simulink subsystem "V2ISimulator"  (R2024a)
settings: Solver=VariableStepAuto  StartTime=0.0  StopTime=10.0  RelTol=1e-3
undefined symbols (not defined in the file or in its folder): SF_std, Ts
settings Model: Creator=The MathWorks, Inc.  LastModifiedBy=L03509110
settings SolverCC: MaxZcPerStep=1
settings DebuggingCC: SubsystemReferenceDiagnosticForUnitTest=warning
settings ModelReferenceCC: EnableRefExpFcnMdlSchedulingChecks=on
settings RTWCC: GPUComputeCapability=3.5  DLArmComputeVersion=19.05

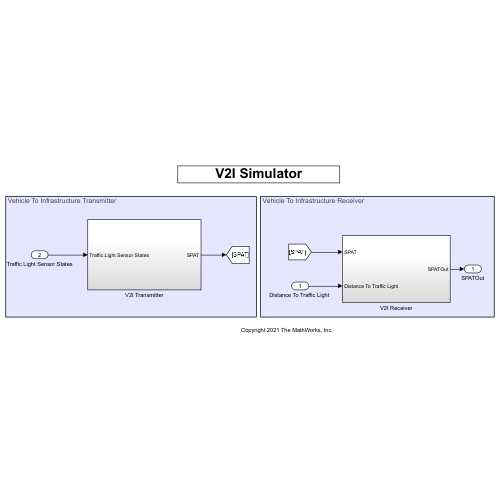
[thumbnail: Simulink's stored preview of the top-level diagram]
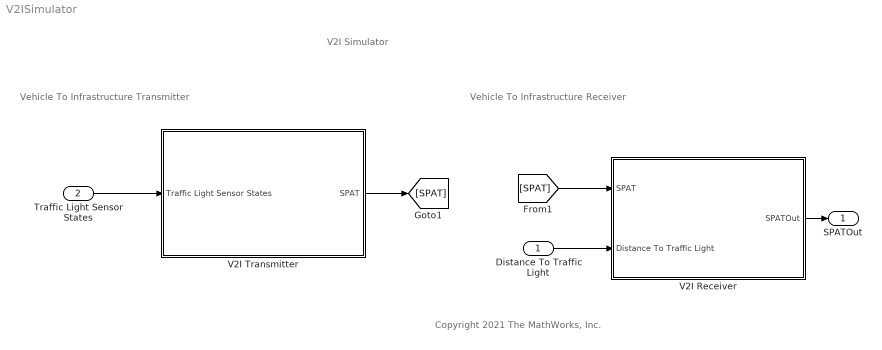
== system V2ISimulator ==
  note: V2I Simulator
  note: Vehicle To Infrastructure Transmitter
  note: Vehicle To Infrastructure Receiver
  note: Copyright 2021 The MathWorks, Inc.
  "Distance To Traffic Light " : Inport
  Traffic Light Sensor States : Inport  Port=2
  V2I Receiver : Subsystem
  V2I Transmitter : Subsystem
  SPATOut : Outport
  wires:
  Traffic Light Sensor States/1 -> V2I Transmitter/1(Traffic Light Sensor States)
  V2I Transmitter/1(SPAT) -> [SPAT]
  V2I Receiver/1(SPATOut) -> SPATOut/1
  "Distance To Traffic Light "/1 -> V2I Receiver/2("Distance To Traffic Light ")
  [SPAT] -> V2I Receiver/1(SPAT)

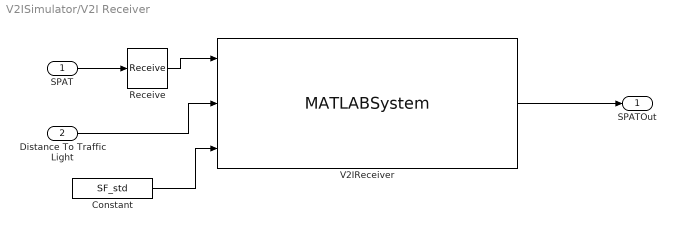
== system V2ISimulator/V2I Receiver ==
  SPAT : Inport  OutDataTypeStr=Bus: BusSPAT  BusOutputAsStruct=on
  "Distance To Traffic Light " : Inport  Port=2
  Constant : Constant  Value=SF_std
  Receive : Receive  InputPortMessageModes=m  UseInternalQueue=off  QueueOverwriting=on  QueueLength=1  QueueType=LIFO
  V2IReceiver : MATLABSystem  System=HelperV2IReceiver  SnrCurves=channelAttributes  OutputStruct=Simulink.Bus.createMATLABStruct('BusSPAT')
      mask Type: HelperV2IReceiver
      mask Display:
      | disp('HelperV2IReceiver');
      | port_label('input',1,'spat');
      | port_label('input',2,'distanceToTrafficLight');
      | port_label('input',3,'SF_std');
      | port_label('output',1,'spatOut');
  SPATOut : Outport
  wires:
  Constant/1 -> V2IReceiver/3
  "Distance To Traffic Light "/1 -> V2IReceiver/2
  SPAT/1 -> Receive/1
  Receive/1 -> V2IReceiver/1
  V2IReceiver/1 -> SPATOut/1

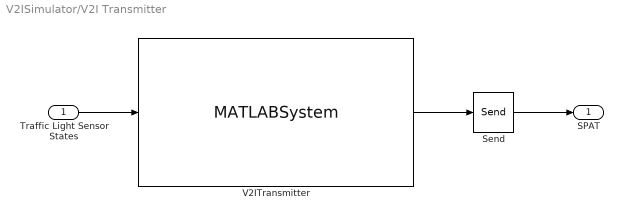
== system V2ISimulator/V2I Transmitter ==
  Traffic Light Sensor States : Inport  PortDimensions=[4 1]  BusOutputAsStruct=on
  Send : Send  OutputPortMessageModes=m
  V2ITransmitter : MATLABSystem  System=V2ITransmitter  RegionInfo=regionInfo  OutputStruct=Simulink.Bus.createMATLABStruct('BusSPAT')
      mask Type: V2ITransmitter
      mask Display:
      | disp('V2ITransmitter');
      | port_label('input',1,'trafficLightStates');
      | port_label('output',1,'spat');
  SPAT : Outport  OutDataTypeStr=Bus: BusSPAT  SampleTime=Ts  BusOutputAsStruct=on
  wires:
  Send/1 -> SPAT/1
  V2ITransmitter/1 -> Send/1
  Traffic Light Sensor States/1 -> V2ITransmitter/1
